simulink model "aeroblk_vmm"  (Simulink 6.0)
settings: Solver=ode45  StartTime=0.0  StopTime=400  FixedStep=0.5
PreLoadFcn:
  | vmm_m=997;vmm_mfuel=399;vmm_Uex=-2700;
  | 
  | vmm_R=0.75;vmm_L=5.5;vmm_Lfuel=0.1341;vmm_Dfuel=1.4671;vmm_rhofuel=1760.4;
  | 
  | vmm_rburn=0.01397;vmm_mmid=237;vmm_mmc=191.2;vmm_mfwd=169.8;vmm_dmid=[2.282 0 0]';
  | 
  | vmm_dmc = [0.067 0 0]'; vmm_dfwd = [4.6975 0 0]';vmm_Lmid=4.2959;vmm_Lmc = 0.1341;vmm_Lfwd = 1.07;
  | 
  | vmm_alt = 0; load aeroblk_vmm_aero;
libraries: simulink x9, aerolibasang x3, aerolibbdyn x3, aerolibanim x1, aerolib6dof2 x1, aerolibadyn x1, aerolibatmos2 x1, aerolibgravity2 x1
CloseFcn:
  | clear vmm_m vmm_mfuel vmm_Uex vmm_R vmm_L vmr_Lfuel vmm_Dfuel vmm_rhofuel vmm_rburn vmm_mmid vmm_mmc vmm_mfwd vmm_dmid vmm_dmc vmm_dfwd vmm_Lmid vmm_Lmc vmm_Lfwd vmm_alt vmm_Lfuel vmm_C*;
  | 
  | h=findobj('type','figure','Name','Animation Figure');if ~isempty(h);close(h);end
settings Model: Creator=The MathWorks Inc.  LastModifiedBy=batserve  ExtModeAutoUpdateStatusClock=off  ProdHWDeviceType=Specified
settings DataIOCC: SaveOutput=off  SaveTime=off  SignalLoggingName=logsOut
settings DebuggingCC: CheckExecutionContextPreStartOutputMsg=on  CheckExecutionContextRuntimeOutputMsg=on  SolverPrmCheckMsg=none
settings HardwareCC: ProdHWDeviceType=Specified

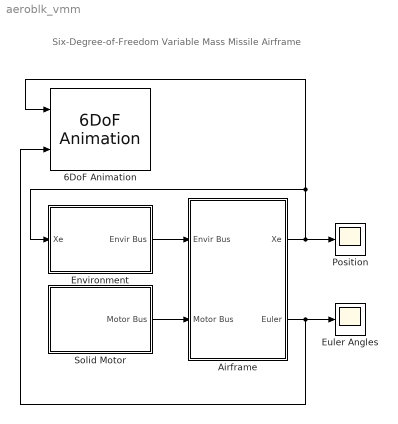
== system aeroblk_vmm ==
  note: Six-Degree-of-Freedom Variable Mass Missile Airframe
  6DoF Animation : aerolibanim/6DoF Animation  u1=[0 2500 -100 1000 -1100 100]  u2=0.2  u3=50.0  u4=[5000 0 5000]  u5=Fly alongside  u6=[50 150 -10]  u7=45  u8=on
  Airframe : Subsystem  PropExecContextAcrossSSBoundary=on
  Environment : Subsystem  PropExecContextAcrossSSBoundary=on
  Euler Angles : Scope
      settings: TimeRange=35  YMin=0  YMax=0.8  SaveName=ScopeData2
  Position : Scope
      settings: TimeRange=35  YMin=-75000  YMax=275000  SaveName=ScopeData3
  Solid Motor : Subsystem  PropExecContextAcrossSSBoundary=on
  wires:
  Environment/1(Envir Bus) -> Airframe/1(Envir Bus)
  Airframe/1(Xe) -> Position/1, 6DoF Animation/1, Environment/1(Xe)
  Airframe/2(Euler) -> Euler Angles/1, 6DoF Animation/2
  Solid Motor/1(Motor Bus) -> Airframe/2(Motor Bus)

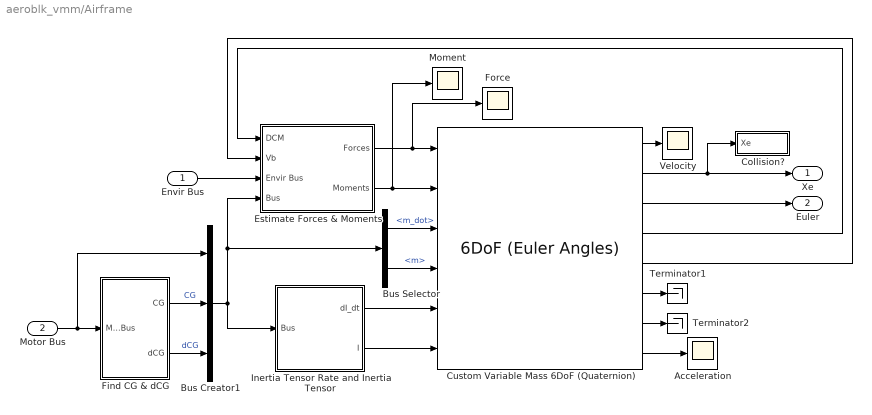
== system aeroblk_vmm/Airframe ==
  Envir Bus : Inport  Port=1  LatchInput=off
  Motor Bus : Inport  Port=2  LatchInput=off
  Acceleration : Scope
      settings: TimeRange=35  YMin=-50  YMax=200
  Bus Creator1 : BusCreator  DialogController=Simulink.DDGSource_Bus  Inputs=3
  Bus Selector : BusSelector  DialogController=Simulink.DDGSource_Bus  OutputSignals=Motor.Propellant.m_dot,Motor.Propellant.m
  Collision? : Subsystem  PropExecContextAcrossSSBoundary=on
  Custom Variable Mass 6DoF (Quaternion) : aerolib6dof2/6DoF (Euler Angles)  units=Metric (MKS)  mtype=Custom Variable  rep=Quaternion  xme_0=[0 0 vmm_alt]  Vm_0=[0 0 0]  eul_0=[0 pi/4 0]  pm_0=[0 0 0]  mass_0=1.0  mass_e=0  mass_f=0  inertia=eye(3)  inertia_e=eye(3)  inertia_f=eye(3)  k_quat=1.0
  Estimate Forces & Moments : Subsystem  PropExecContextAcrossSSBoundary=on
  Find CG & dCG : Subsystem  PropExecContextAcrossSSBoundary=on
  Force : Scope
      settings: TimeRange=35  YMin=-20000  YMax=120000  SaveName=ScopeData7
  Inertia Tensor Rate and Inertia Tensor : Subsystem  PropExecContextAcrossSSBoundary=on
  Moment : Scope
      settings: TimeRange=35  YMin=-40000  YMax=60000  SaveName=ScopeData4
  Terminator1 : Terminator
  Terminator2 : Terminator
  Velocity : Scope
      settings: TimeRange=35  YMin=-150  YMax=150
  Xe : Outport
  Euler : Outport  Port=2
  wires:
  Motor Bus/1 -> Bus Creator1/1, Find CG & dCG/1(Motor Bus)
  Bus Creator1/1 -> Inertia Tensor Rate and Inertia Tensor/1(Bus), Bus Selector/1, Estimate Forces & Moments/4(Bus)
  Find CG & dCG/1(CG) -> Bus Creator1/2  "CG"
  Find CG & dCG/2(dCG) -> Bus Creator1/3  "dCG"
  Estimate Forces & Moments/1(Forces) -> Force/1, Custom Variable Mass 6DoF (Quaternion)/1
  Bus Selector/2 -> Custom Variable Mass 6DoF (Quaternion)/4  "<m>"
  Bus Selector/1 -> Custom Variable Mass 6DoF (Quaternion)/3  "<m_dot>"
  Custom Variable Mass 6DoF (Quaternion)/2 -> Xe/1, Collision?/1(Xe)
  Inertia Tensor Rate and Inertia Tensor/1(dI_dt) -> Custom Variable Mass 6DoF (Quaternion)/5
  Inertia Tensor Rate and Inertia Tensor/2(I) -> Custom Variable Mass 6DoF (Quaternion)/6
  Custom Variable Mass 6DoF (Quaternion)/3 -> Euler/1
  Custom Variable Mass 6DoF (Quaternion)/7 -> Terminator2/1
  Custom Variable Mass 6DoF (Quaternion)/6 -> Terminator1/1
  Custom Variable Mass 6DoF (Quaternion)/5 -> Estimate Forces & Moments/2(Vb)
  Custom Variable Mass 6DoF (Quaternion)/4 -> Estimate Forces & Moments/1(DCM)
  Custom Variable Mass 6DoF (Quaternion)/1 -> Velocity/1
  Custom Variable Mass 6DoF (Quaternion)/8 -> Acceleration/1
  Estimate Forces & Moments/2(Moments) -> Moment/1, Custom Variable Mass 6DoF (Quaternion)/2
  Envir Bus/1 -> Estimate Forces & Moments/3(Envir Bus)

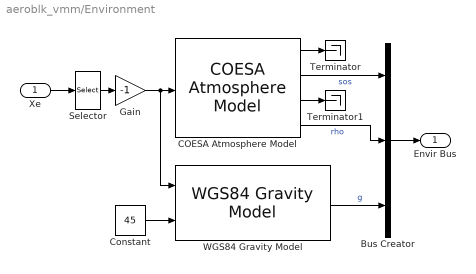
== system aeroblk_vmm/Environment ==
  Xe : Inport  Port=1  LatchInput=off
  Bus Creator : BusCreator  DialogController=Simulink.DDGSource_Bus  Inputs=3
  COESA Atmosphere Model : aerolibatmos2/COESA Atmosphere Model  units=Metric (MKS)  spec=1976 COESA-extended U.S. Standard Atmosphere  model=Profile  profile_var=High temperature  profile_percent=1%  profile_alt=5 km (16404 ft)  envelope_var=High temperature  envelope_percent=1%  action=None
  Constant : Constant  Value=45
  Gain : Gain  Gain=-1  SaturateOnIntegerOverflow=on
  Selector : Selector  Elements=3  InputPortWidth=3
  Terminator : Terminator
  Terminator1 : Terminator
  WGS84 Gravity Model : aerolibgravity2/WGS84 Gravity Model  model=WGS84 Taylor Series  units=Metric (MKS)  no_atmos=on  precessing=on  month=February  day=1  year=2000  no_centrifugal=on  action=None
  Envir Bus : Outport
  wires:
  Selector/1 -> Gain/1
  Gain/1 -> COESA Atmosphere Model/1, WGS84 Gravity Model/1
  Xe/1 -> Selector/1
  COESA Atmosphere Model/1 -> Terminator/1
  COESA Atmosphere Model/2 -> Bus Creator/1  "sos"
  COESA Atmosphere Model/3 -> Terminator1/1
  COESA Atmosphere Model/4 -> Bus Creator/2  "rho"
  WGS84 Gravity Model/1 -> Bus Creator/3  "g"
  Constant/1 -> WGS84 Gravity Model/2
  Bus Creator/1 -> Envir Bus/1

== system aeroblk_vmm/Solid Motor ==
  note: *Assume steady burning and steady flow conditions
      |   dMass/dt = 1/4\rho\pid^2r_{burn}
      | *Assume end burning propellent -neutral burning
  "Find dm/dt, m,  CG & L" : Subsystem  PropExecContextAcrossSSBoundary=on
  Propellent Burn Rate : Constant  Value=vmm_rburn
  Propellent Density : Constant  Value=vmm_rhofuel
  Propellent Diameter : Constant  Value=vmm_Dfuel
  Motor Bus : Outport
  wires:
  Propellent Diameter/1 -> "Find dm/dt, m,  CG & L"/2(diameter)
  Propellent Density/1 -> "Find dm/dt, m,  CG & L"/1(density)
  Propellent Burn Rate/1 -> "Find dm/dt, m,  CG & L"/3(burn rate)
  "Find dm/dt, m,  CG & L"/1(Bus) -> Motor Bus/1  "Motor"

== system aeroblk_vmm/Airframe/Collision? ==
  Xe : Inport  Port=1  LatchInput=off
  Check Static  Upper Bound : simulink/Model Verification/Check Static  Upper Bound  Description=u <= vmm_alt  max=vmm_alt  max_included=on  enabled=on  callback=disp('Collision with ground')  stopWhenAssertionFail=off  export=on  icon=graphic
  Logical Operator : Logic  Operator=NOT  AllPortsSameDT=off
  Selector : Selector  Elements=3  InputPortWidth=3
  Stop Simulation : Stop
  wires:
  Selector/1 -> Check Static  Upper Bound/1
  Check Static  Upper Bound/1 -> Logical Operator/1
  Logical Operator/1 -> Stop Simulation/1
  Xe/1 -> Selector/1

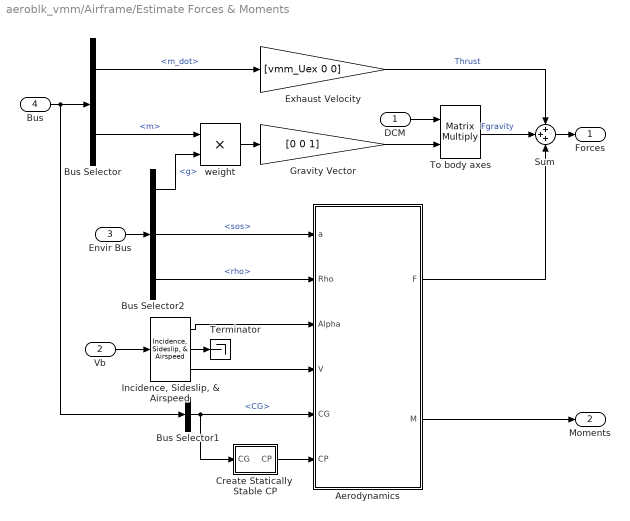
== system aeroblk_vmm/Airframe/Estimate Forces & Moments ==
  DCM : Inport  Port=1  LatchInput=off
  Vb : Inport  Port=2  LatchInput=off
  Envir Bus : Inport  Port=3  LatchInput=off
  Bus : Inport  Port=4  LatchInput=off
  Aerodynamics : Subsystem  PropExecContextAcrossSSBoundary=on
  Bus Selector : BusSelector  DialogController=Simulink.DDGSource_Bus  OutputSignals=Motor.Propellant.m_dot,Motor.Propellant.m
  Bus Selector1 : BusSelector  DialogController=Simulink.DDGSource_Bus  OutputSignals=CG
  Bus Selector2 : BusSelector  DialogController=Simulink.DDGSource_Bus  OutputSignals=g,sos,rho
  Create Statically  Stable CP : Subsystem  PropExecContextAcrossSSBoundary=on
  Exhaust Velocity : Gain  Gain=[vmm_Uex 0 0]
  Gravity Vector : Gain  Gain=[0 0 1]
  "Incidence, Sideslip, & Airspeed" : aerolibasang/Incidence, Sideslip, & Airspeed
  Sum : Sum  Inputs=+++  SaturateOnIntegerOverflow=on
  Terminator : Terminator
  To body axes : Product  Multiplication=Matrix(*)  SaturateOnIntegerOverflow=on
  weight : Product  SaturateOnIntegerOverflow=on
  Forces : Outport
  Moments : Outport  Port=2
  wires:
  Gravity Vector/1 -> To body axes/2
  Exhaust Velocity/1 -> Sum/1  "Thrust"
  DCM/1 -> To body axes/1
  To body axes/1 -> Sum/2  "Fgravity"
  Bus Selector/2 -> weight/1  "<m>"
  Bus Selector/1 -> Exhaust Velocity/1  "<m_dot>"
  Bus/1 -> Bus Selector/1, Bus Selector1/1
  Sum/1 -> Forces/1
  Aerodynamics/2(" M") -> Moments/1
  Aerodynamics/1(F) -> Sum/3
  Envir Bus/1 -> Bus Selector2/1
  Bus Selector2/2 -> Aerodynamics/1(a)  "<sos>"
  Bus Selector2/3 -> Aerodynamics/2(Rho)  "<rho>"
  Vb/1 -> "Incidence, Sideslip, & Airspeed"/1
  "Incidence, Sideslip, & Airspeed"/1 -> Aerodynamics/3(Alpha)
  "Incidence, Sideslip, & Airspeed"/3 -> Aerodynamics/4(V)
  "Incidence, Sideslip, & Airspeed"/2 -> Terminator/1
  Bus Selector2/1 -> weight/2  "<g>"
  weight/1 -> Gravity Vector/1
  Bus Selector1/1 -> Aerodynamics/5(CG), Create Statically  Stable CP/1(CG)  "<CG>"
  Create Statically  Stable CP/1(CP) -> Aerodynamics/6(CP)

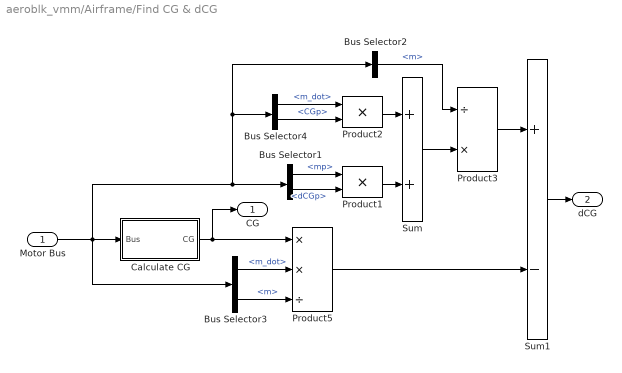
== system aeroblk_vmm/Airframe/Find CG & dCG ==
  Motor Bus : Inport  Port=1  LatchInput=off
  Bus Selector1 : BusSelector  DialogController=Simulink.DDGSource_Bus  OutputSignals=mp,dCGp
  Bus Selector2 : BusSelector  DialogController=Simulink.DDGSource_Bus  OutputSignals=Propellant.m
  Bus Selector3 : BusSelector  DialogController=Simulink.DDGSource_Bus  OutputSignals=Propellant.m_dot,Propellant.m
  Bus Selector4 : BusSelector  DialogController=Simulink.DDGSource_Bus  OutputSignals=Propellant.m_dot,CGp
  Calculate CG : Subsystem  PropExecContextAcrossSSBoundary=on
  Product1 : Product  SaturateOnIntegerOverflow=on
  Product2 : Product  SaturateOnIntegerOverflow=on
  Product3 : Product  Inputs=/*  SaturateOnIntegerOverflow=on
  Product5 : Product  Inputs=**/  SaturateOnIntegerOverflow=on
  Sum : Sum  Inputs=2  SaturateOnIntegerOverflow=on
  Sum1 : Sum  Inputs=+-  SaturateOnIntegerOverflow=on
  CG : Outport
  dCG : Outport  Port=2
  wires:
  Bus Selector3/2 -> Product5/3  "<m>"
  Bus Selector3/1 -> Product5/2  "<m_dot>"
  Bus Selector2/1 -> Product3/1  "<m>"
  Sum1/1 -> dCG/1
  Product3/1 -> Sum1/1
  Sum/1 -> Product3/2
  Product5/1 -> Sum1/2
  Product1/1 -> Sum/2
  Product2/1 -> Sum/1
  Calculate CG/1(CG) -> CG/1, Product5/1
  Motor Bus/1 -> Bus Selector3/1, Calculate CG/1(Bus), Bus Selector2/1, Bus Selector4/1, Bus Selector1/1
  Bus Selector1/1 -> Product1/1  "<mp>"
  Bus Selector1/2 -> Product1/2  "<dCGp>"
  Bus Selector4/1 -> Product2/1  "<m_dot>"
  Bus Selector4/2 -> Product2/2  "<CGp>"

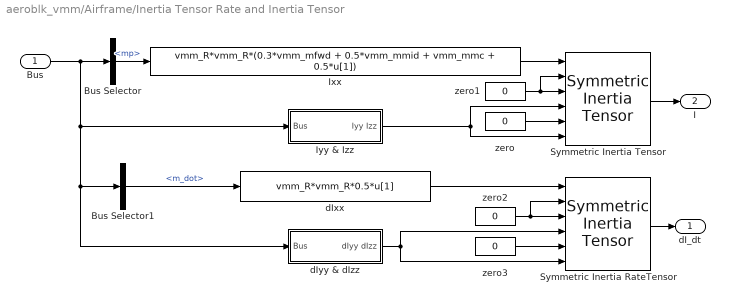
== system aeroblk_vmm/Airframe/Inertia Tensor Rate and Inertia Tensor ==
  Bus : Inport  Port=1  LatchInput=off
  Bus Selector : BusSelector  DialogController=Simulink.DDGSource_Bus  OutputSignals=Motor.mp
  Bus Selector1 : BusSelector  DialogController=Simulink.DDGSource_Bus  OutputSignals=Motor.Propellant.m_dot
  Ixx : Fcn  Expr=vmm_R*vmm_R*(0.3*vmm_mfwd + 0.5*vmm_mmid + vmm_mmc + 0.5*u[1])
  Iyy & Izz : Subsystem  PropExecContextAcrossSSBoundary=on
  Symmetric Inertia RateTensor : aerolibbdyn/Symmetric Inertia Tensor
  Symmetric Inertia Tensor : aerolibbdyn/Symmetric Inertia Tensor
  dIxx : Fcn  Expr=vmm_R*vmm_R*0.5*u[1]
  dIyy & dIzz : Subsystem  PropExecContextAcrossSSBoundary=on
  zero{,1..3} (4 alike) : Constant  Value=0
  dI_dt : Outport
  I : Outport  Port=2
  wires:
  Symmetric Inertia RateTensor/1 -> dI_dt/1
  Bus/1 -> Bus Selector/1, Iyy & Izz/1(Bus), Bus Selector1/1, dIyy & dIzz/1(Bus)
  Ixx/1 -> Symmetric Inertia Tensor/1
  Iyy & Izz/1(Iyy Izz) -> Symmetric Inertia Tensor/6, Symmetric Inertia Tensor/4
  Symmetric Inertia Tensor/1 -> I/1
  Bus Selector/1 -> Ixx/1  "<mp>"
  zero/1 -> Symmetric Inertia Tensor/5
  zero1/1 -> Symmetric Inertia Tensor/2, Symmetric Inertia Tensor/3
  Bus Selector1/1 -> dIxx/1  "<m_dot>"
  dIxx/1 -> Symmetric Inertia RateTensor/1
  zero2/1 -> Symmetric Inertia RateTensor/2, Symmetric Inertia RateTensor/3
  dIyy & dIzz/1(dIyy dIzz) -> Symmetric Inertia RateTensor/4, Symmetric Inertia RateTensor/6
  zero3/1 -> Symmetric Inertia RateTensor/5

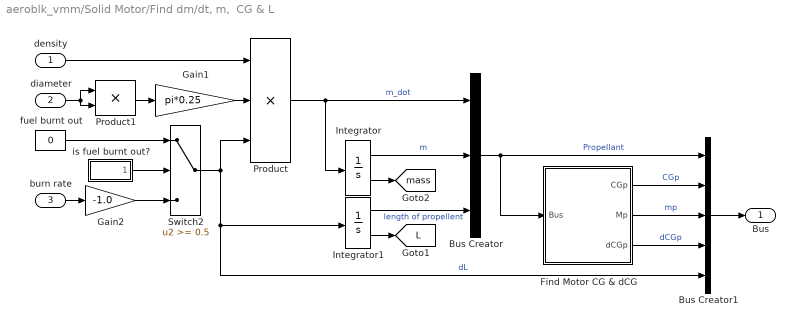
== system aeroblk_vmm/Solid Motor/Find dm/dt, m,  CG & L ==
  density : Inport  Port=1  LatchInput=off
  diameter : Inport  Port=2  LatchInput=off
  burn rate : Inport  Port=3  LatchInput=off
  Bus Creator : BusCreator  DialogController=Simulink.DDGSource_Bus  Inputs=3
  Bus Creator1 : BusCreator  DialogController=Simulink.DDGSource_Bus  Inputs=5
  Find Motor CG & dCG : Subsystem  PropExecContextAcrossSSBoundary=on
  Gain1 : Gain  Gain=pi*0.25  SaturateOnIntegerOverflow=on
  Gain2 : Gain  Gain=-1.0  SaturateOnIntegerOverflow=on
  Integrator : Integrator  InitialCondition=vmm_m  LimitOutput=on  UpperSaturationLimit=vmm_m  LowerSaturationLimit=vmm_m-vmm_mfuel  ShowSaturationPort=on
  Integrator1 : Integrator  InitialCondition=vmm_Lfuel  LimitOutput=on  UpperSaturationLimit=vmm_Lfuel  LowerSaturationLimit=0  ShowSaturationPort=on
  Product : Product  Inputs=3  SaturateOnIntegerOverflow=on
  Product1 : Product  SaturateOnIntegerOverflow=on
  Switch2 : Switch  Threshold=0.5  SaturateOnIntegerOverflow=on  InputSameDT=on
  fuel burnt out : Constant  Value=0
  is fuel burnt out? : Subsystem  PropExecContextAcrossSSBoundary=on
  Bus : Outport
  tag scope: L=global, mass=global
  wires:
  Integrator/2 -> [mass]
  Product/1 -> Integrator/1, Bus Creator/1  "m_dot"
  Integrator/1 -> Bus Creator/2  "m"
  density/1 -> Product/1
  diameter/1 -> Product1/1, Product1/2
  burn rate/1 -> Gain2/1
  Integrator1/1 -> Bus Creator/3  "length of propellent"
  Bus Creator/1 -> Bus Creator1/1, Find Motor CG & dCG/1(Bus)  "Propellant"
  Find Motor CG & dCG/1(CGp) -> Bus Creator1/2  "CGp"
  Bus Creator1/1 -> Bus/1
  Find Motor CG & dCG/3(dCGp) -> Bus Creator1/4  "dCGp"
  Product1/1 -> Gain1/1
  Gain1/1 -> Product/2
  Gain2/1 -> Switch2/3
  fuel burnt out/1 -> Switch2/1
  Integrator1/2 -> [L]
  Switch2/1 -> Product/3, Integrator1/1, Bus Creator1/5  "dL"
  is fuel burnt out?/1(switch) -> Switch2/2
  Find Motor CG & dCG/2(Mp) -> Bus Creator1/3  "mp"

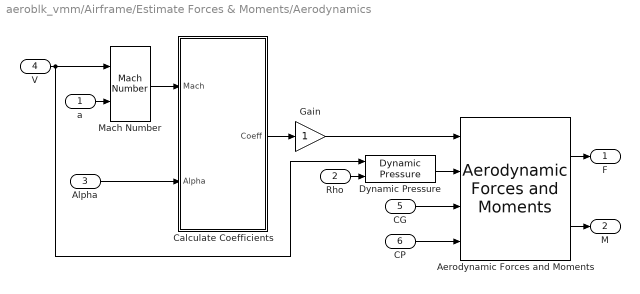
== system aeroblk_vmm/Airframe/Estimate Forces & Moments/Aerodynamics ==
  a : Inport  Port=1  LatchInput=off
  Rho : Inport  Port=2  LatchInput=off
  Alpha : Inport  Port=3  LatchInput=off
  V : Inport  Port=4  LatchInput=off
  CG : Inport  Port=5  LatchInput=off
  CP : Inport  Port=6  LatchInput=off
  Aerodynamic Forces and Moments : aerolibadyn/Aerodynamic Forces and Moments  S=pi*vmm_R*vmm_R  b=2*vmm_R  cbar=2*vmm_R
  Calculate Coefficients : Subsystem  PropExecContextAcrossSSBoundary=on
  Dynamic Pressure : aerolibasang/Dynamic Pressure
  Gain : Gain  SaturateOnIntegerOverflow=on
  Mach Number : aerolibasang/Mach Number
  F : Outport  InitialOutput=[0]
  " M" : Outport  Port=2  InitialOutput=0
  wires:
  Mach Number/1 -> Calculate Coefficients/1(Mach)
  Alpha/1 -> Calculate Coefficients/2(Alpha)
  a/1 -> Mach Number/2
  V/1 -> Mach Number/1, Dynamic Pressure/1
  Dynamic Pressure/1 -> Aerodynamic Forces and Moments/2
  Rho/1 -> Dynamic Pressure/2
  CG/1 -> Aerodynamic Forces and Moments/3
  CP/1 -> Aerodynamic Forces and Moments/4
  Aerodynamic Forces and Moments/1 -> F/1
  Aerodynamic Forces and Moments/2 -> " M"/1
  Calculate Coefficients/1(Coeff) -> Gain/1
  Gain/1 -> Aerodynamic Forces and Moments/1

== system aeroblk_vmm/Airframe/Estimate Forces & Moments/Create Statically  Stable CP ==
  CG : Inport  Port=1  LatchInput=off
  Constant : Constant  Value=0.1
  Sum1 : Sum  Inputs=|+-  SaturateOnIntegerOverflow=on
  CP : Outport
  wires:
  Constant/1 -> Sum1/2
  CG/1 -> Sum1/1
  Sum1/1 -> CP/1

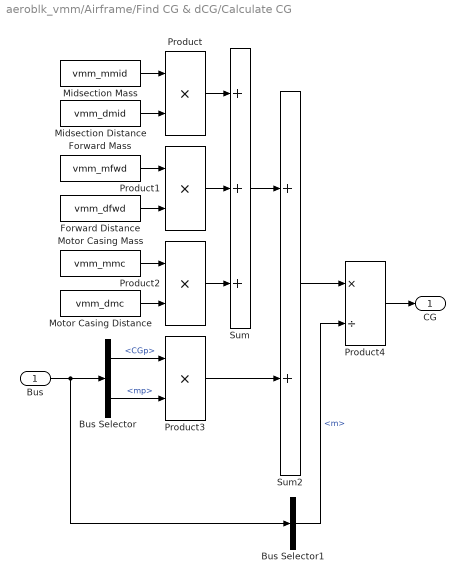
== system aeroblk_vmm/Airframe/Find CG & dCG/Calculate CG ==
  Bus : Inport  Port=1  LatchInput=off
  Bus Selector : BusSelector  DialogController=Simulink.DDGSource_Bus  OutputSignals=CGp,mp
  Bus Selector1 : BusSelector  DialogController=Simulink.DDGSource_Bus  OutputSignals=Propellant.m
  Forward Distance : Constant  Value=vmm_dfwd
  Forward Mass : Constant  Value=vmm_mfwd
  Midsection Distance : Constant  Value=vmm_dmid
  Midsection Mass : Constant  Value=vmm_mmid
  Motor Casing Distance : Constant  Value=vmm_dmc
  Motor Casing Mass : Constant  Value=vmm_mmc
  Product{,1..3} (4 alike) : Product  SaturateOnIntegerOverflow=on
  Product4 : Product  Inputs=*/  SaturateOnIntegerOverflow=on
  Sum : Sum  Inputs=3  SaturateOnIntegerOverflow=on
  Sum2 : Sum  Inputs=2  SaturateOnIntegerOverflow=on
  CG : Outport
  wires:
  Product4/1 -> CG/1
  Sum2/1 -> Product4/1
  Midsection Distance/1 -> Product/2
  Midsection Mass/1 -> Product/1
  Forward Distance/1 -> Product1/2
  Forward Mass/1 -> Product1/1
  Motor Casing Distance/1 -> Product2/2
  Motor Casing Mass/1 -> Product2/1
  Product/1 -> Sum/1
  Product1/1 -> Sum/2
  Product2/1 -> Sum/3
  Product3/1 -> Sum2/2
  Sum/1 -> Sum2/1
  Bus Selector/2 -> Product3/2  "<mp>"
  Bus/1 -> Bus Selector1/1, Bus Selector/1
  Bus Selector1/1 -> Product4/2  "<m>"
  Bus Selector/1 -> Product3/1  "<CGp>"

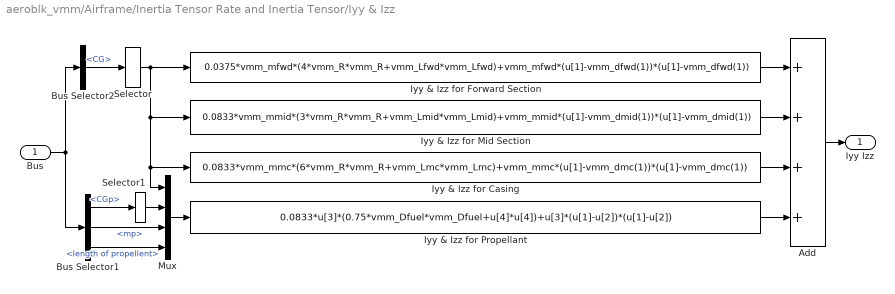
== system aeroblk_vmm/Airframe/Inertia Tensor Rate and Inertia Tensor/Iyy & Izz ==
  Bus : Inport  Port=1  LatchInput=off
  Add : Sum  Inputs=++++  OutScaling=2^-10
  Bus Selector1 : BusSelector  DialogController=Simulink.DDGSource_Bus  OutputSignals=Motor.CGp,Motor.mp,Motor.Propellant.length of propellent
  Bus Selector2 : BusSelector  DialogController=Simulink.DDGSource_Bus  OutputSignals=CG
  Iyy & Izz for Casing : Fcn  Expr=0.0833*vmm_mmc*(6*vmm_R*vmm_R+vmm_Lmc*vmm_Lmc)+vmm_mmc*(u[1]-vmm_dmc(1))*(u[1]-vmm_dmc(1))
  Iyy & Izz for Forward Section : Fcn  Expr=0.0375*vmm_mfwd*(4*vmm_R*vmm_R+vmm_Lfwd*vmm_Lfwd)+vmm_mfwd*(u[1]-vmm_dfwd(1))*(u[1]-vmm_dfwd(1))
  Iyy & Izz for Mid Section : Fcn  Expr=0.0833*vmm_mmid*(3*vmm_R*vmm_R+vmm_Lmid*vmm_Lmid)+vmm_mmid*(u[1]-vmm_dmid(1))*(u[1]-vmm_dmid(1))
  Iyy & Izz for Propellant : Fcn  Expr=0.0833*u[3]*(0.75*vmm_Dfuel*vmm_Dfuel+u[4]*u[4])+u[3]*(u[1]-u[2])*(u[1]-u[2])
  Mux : Mux
  Selector : Selector  InputPortWidth=3
  Selector1 : Selector  InputPortWidth=3
  Iyy Izz : Outport
  wires:
  Iyy & Izz for Forward Section/1 -> Add/1
  Iyy & Izz for Mid Section/1 -> Add/2
  Iyy & Izz for Casing/1 -> Add/3
  Iyy & Izz for Propellant/1 -> Add/4
  Add/1 -> Iyy Izz/1
  Selector/1 -> Iyy & Izz for Forward Section/1, Iyy & Izz for Mid Section/1, Iyy & Izz for Casing/1, Mux/1
  Mux/1 -> Iyy & Izz for Propellant/1
  Bus/1 -> Bus Selector1/1, Bus Selector2/1
  Bus Selector1/1 -> Selector1/1  "<CGp>"
  Bus Selector2/1 -> Selector/1  "<CG>"
  Bus Selector1/2 -> Mux/3  "<mp>"
  Bus Selector1/3 -> Mux/4  "<length of propellent>"
  Selector1/1 -> Mux/2

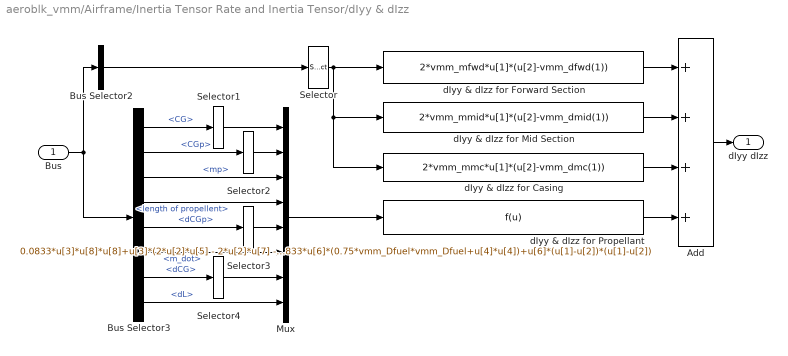
== system aeroblk_vmm/Airframe/Inertia Tensor Rate and Inertia Tensor/dIyy & dIzz ==
  Bus : Inport  Port=1  LatchInput=off
  Add : Sum  Inputs=++++  OutScaling=2^-10
  Bus Selector2 : BusSelector  DialogController=Simulink.DDGSource_Bus  OutputSignals=dCG,CG  MuxedOutput=on
  Bus Selector3 : BusSelector  DialogController=Simulink.DDGSource_Bus  OutputSignals=CG,Motor.CGp,Motor.mp,Motor.Propellant.length of propellent,Motor.dCGp,Motor.Propellant.m_dot,dCG,Motor.dL
  Mux : Mux  Inputs=8
  Selector : Selector  Elements=[1 4]  InputPortWidth=6
  Selector{1..4} (4 alike) : Selector  InputPortWidth=3
  dIyy & dIzz for Casing : Fcn  Expr=2*vmm_mmc*u[1]*(u[2]-vmm_dmc(1))
  dIyy & dIzz for Forward Section : Fcn  Expr=2*vmm_mfwd*u[1]*(u[2]-vmm_dfwd(1))
  dIyy & dIzz for Mid Section : Fcn  Expr=2*vmm_mmid*u[1]*(u[2]-vmm_dmid(1))
  dIyy & dIzz for Propellant : Fcn  Expr=0.0833*u[3]*u[8]*u[8]+u[3]*(2*u[2]*u[5] - 2*u[2]*u[7] -2*u[5]*u[1] + 2*u[1]*u[7]) + 0.0833*u[6]*(0.75*vmm_Dfuel*vmm_Dfuel+u[4]*u[4])+u[6]*(u[1]-u[2])*(u[1]-u[2])
  dIyy dIzz : Outport
  wires:
  Bus Selector2/1 -> Selector/1
  Bus/1 -> Bus Selector2/1, Bus Selector3/1
  Selector/1 -> dIyy & dIzz for Mid Section/1, dIyy & dIzz for Casing/1, dIyy & dIzz for Forward Section/1
  Add/1 -> dIyy dIzz/1
  dIyy & dIzz for Propellant/1 -> Add/4
  dIyy & dIzz for Casing/1 -> Add/3
  dIyy & dIzz for Mid Section/1 -> Add/2
  dIyy & dIzz for Forward Section/1 -> Add/1
  Bus Selector3/2 -> Selector2/1  "<CGp>"
  Bus Selector3/5 -> Selector3/1  "<dCGp>"
  Bus Selector3/7 -> Selector4/1  "<dCG>"
  Selector2/1 -> Mux/2
  Bus Selector3/3 -> Mux/3  "<mp>"
  Bus Selector3/4 -> Mux/4  "<length of propellent>"
  Selector3/1 -> Mux/5
  Bus Selector3/6 -> Mux/6  "<m_dot>"
  Selector4/1 -> Mux/7
  Bus Selector3/8 -> Mux/8  "<dL>"
  Bus Selector3/1 -> Selector1/1  "<CG>"
  Selector1/1 -> Mux/1
  Mux/1 -> dIyy & dIzz for Propellant/1

== system aeroblk_vmm/Solid Motor/Find dm/dt, m,  CG & L/Find Motor CG & dCG ==
  Bus : Inport  Port=1  LatchInput=off
  Bus Selector : BusSelector  DialogController=Simulink.DDGSource_Bus  OutputSignals=m,m_dot
  Bus Selector1 : BusSelector  DialogController=Simulink.DDGSource_Bus  OutputSignals=m
  Estimate Center of Gravity : aerolibbdyn/Estimate Center of Gravity  fmass=vmm_m  emass=vmm_m-vmm_mfuel  fcg=[vmm_Lfuel*0.5 0 0]'  ecg=[vmm_Lfuel 0 0]'
  Fixed Missile Mass : Constant  Value=vmm_m-vmm_mfuel
  Sum1 : Sum  Inputs=|-+  SaturateOnIntegerOverflow=on
  CGp : Outport
  Mp : Outport  Port=2
  dCGp : Outport  Port=3
  wires:
  Estimate Center of Gravity/1 -> CGp/1
  Sum1/1 -> Mp/1
  Estimate Center of Gravity/2 -> dCGp/1
  Bus Selector/1 -> Estimate Center of Gravity/1  "<m>"
  Bus Selector/2 -> Estimate Center of Gravity/2  "<m_dot>"
  Bus/1 -> Bus Selector/1, Bus Selector1/1
  Bus Selector1/1 -> Sum1/2  "<m>"
  Fixed Missile Mass/1 -> Sum1/1

== system aeroblk_vmm/Solid Motor/Find dm/dt, m,  CG & L/is fuel burnt out? ==
  0.5 : Constant  Value=-0.5
  Logical Operator : Logic  Operator=OR  Inputs=1  AllPortsSameDT=off  OutDataTypeMode=Boolean
  Mux : Mux  Inputs=2
  Relational Operator : RelationalOperator  Operator=<
  switch : Outport
  wires:
  [L] -> Mux/2
  0.5/1 -> Relational Operator/2
  Relational Operator/1 -> Logical Operator/1
  [mass] -> Mux/1
  Mux/1 -> Relational Operator/1
  Logical Operator/1 -> switch/1

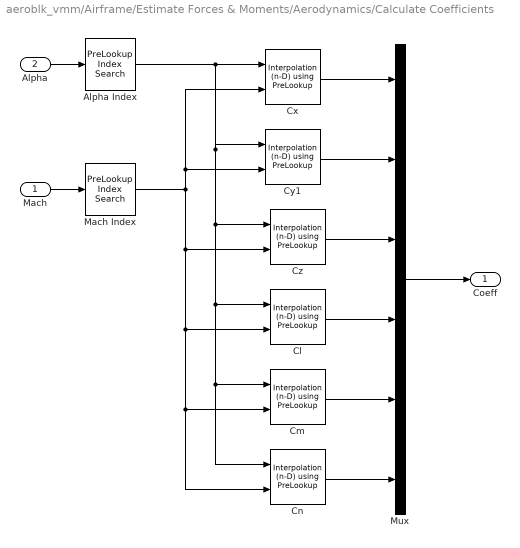
== system aeroblk_vmm/Airframe/Estimate Forces & Moments/Aerodynamics/Calculate Coefficients ==
  Mach : Inport  Port=1  LatchInput=off
  Alpha : Inport  Port=2  LatchInput=off
  Alpha Index : simulink/Lookup Tables/PreLookup Index Search  bpData=vmm_Calpha  searchMode=Binary Search  cacheBpFlag=on  outputFlag=off  IndexDataType=uint32  extrapMode=Linear Extrapolation  rangeErrorMode=None
  Cl : simulink/Lookup Tables/Interpolation (n-D) using PreLookup  numDimsPopupSelect=2  explicitNumDims=2  table=vmm_CLB'  interpMethod=Linear  extrapMethod=Linear  rangeErrorMode=None  NumSelectionDims=0
  Cm : simulink/Lookup Tables/Interpolation (n-D) using PreLookup  numDimsPopupSelect=2  explicitNumDims=2  table=vmm_CM'  interpMethod=Linear  extrapMethod=Linear  rangeErrorMode=None  NumSelectionDims=0
  Cn : simulink/Lookup Tables/Interpolation (n-D) using PreLookup  numDimsPopupSelect=2  explicitNumDims=2  table=vmm_CNB'  interpMethod=Linear  extrapMethod=Linear  rangeErrorMode=None  NumSelectionDims=0
  Cx : simulink/Lookup Tables/Interpolation (n-D) using PreLookup  numDimsPopupSelect=2  explicitNumDims=2  table=vmm_CX'  interpMethod=Linear  extrapMethod=Linear  rangeErrorMode=None  NumSelectionDims=0
  Cy1 : simulink/Lookup Tables/Interpolation (n-D) using PreLookup  numDimsPopupSelect=2  explicitNumDims=2  table=vmm_CY'  interpMethod=Linear  extrapMethod=Linear  rangeErrorMode=None  NumSelectionDims=0
  Cz : simulink/Lookup Tables/Interpolation (n-D) using PreLookup  numDimsPopupSelect=2  explicitNumDims=2  table=vmm_CZ'  interpMethod=Linear  extrapMethod=Linear  rangeErrorMode=None  NumSelectionDims=0
  Mach Index : simulink/Lookup Tables/PreLookup Index Search  bpData=vmm_CMach  searchMode=Binary Search  cacheBpFlag=on  outputFlag=off  IndexDataType=uint32  extrapMode=Linear Extrapolation  rangeErrorMode=None
  Mux : Mux  Inputs=6
  Coeff : Outport  InitialOutput=0
  wires:
  Mach/1 -> Mach Index/1
  Alpha/1 -> Alpha Index/1
  Cm/1 -> Mux/5
  Cz/1 -> Mux/3
  Cx/1 -> Mux/1
  Mach Index/1 -> Cz/2, Cm/2, Cn/2, Cl/2, Cx/2, Cy1/2
  Alpha Index/1 -> Cm/1, Cn/1, Cl/1, Cz/1, Cy1/1, Cx/1
  Cn/1 -> Mux/6
  Cy1/1 -> Mux/2
  Cl/1 -> Mux/4
  Mux/1 -> Coeff/1
